simulink subsystem "Distance_from_Speaker"  (R2023b)
settings: Solver=VariableStepAuto  StartTime=0.0  StopTime=10.0  RelTol=1e-3
undefined symbols (not defined in the file): AT_Tag_4_Coordinate_X, AT_Tag_4_Coordinate_Y, AT_Tag_7_Coordinate_X, AT_Tag_7_Coordinate_Y, KF_Vision_Ambiguity_Thresh
libraries: simulink x1
settings Model: Creator=ander  LastModifiedBy=ander

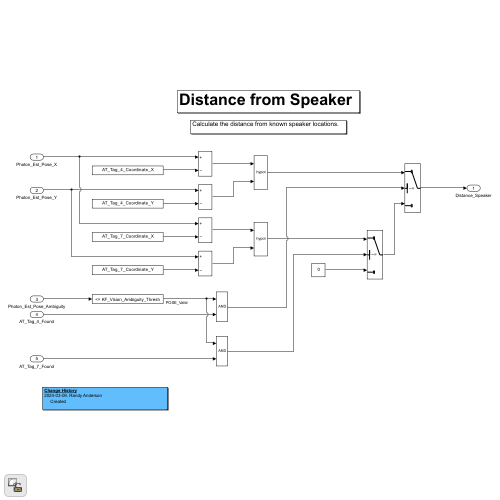
[thumbnail: Simulink's stored preview of the top-level diagram]
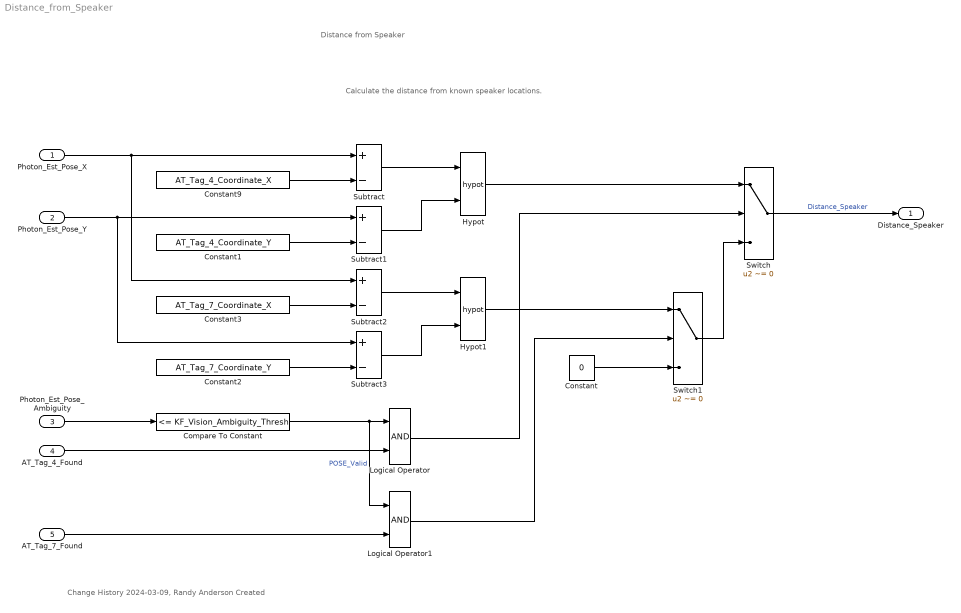
== system Distance_from_Speaker ==
  note: Distance from Speaker
  note: Calculate the distance from known speaker locations.
  note: Change History
      | 2024-03-09, Randy Anderson
      | Created
  Photon_Est_Pose_X : Inport
  Photon_Est_Pose_Y : Inport  Port=2
  Photon_Est_Pose_Ambiguity : Inport  Port=3
  AT_Tag_4_Found : Inport  Port=4
  AT_Tag_7_Found : Inport  Port=5
  Compare To Constant : simulink/Logic and Bit Operations/Compare To Constant  relop=<=  const=KF_Vision_Ambiguity_Thresh  OutDataTypeStr=boolean
  Constant : Constant  Value=0
  Constant1 : Constant  Value=AT_Tag_4_Coordinate_Y
  Constant2 : Constant  Value=AT_Tag_7_Coordinate_Y
  Constant3 : Constant  Value=AT_Tag_7_Coordinate_X
  Constant9 : Constant  Value=AT_Tag_4_Coordinate_X
  Hypot : Math  Operator=hypot
  Hypot1 : Math  Operator=hypot
  Logical Operator : Logic  AllPortsSameDT=off  OutDataTypeStr=boolean
  Logical Operator1 : Logic  AllPortsSameDT=off  OutDataTypeStr=boolean
  Subtract{,1..3} (4 alike) : Sum  Inputs=+-
  Switch : Switch  Criteria=u2 ~= 0  SaturateOnIntegerOverflow=off  InputSameDT=off
  Switch1 : Switch  Criteria=u2 ~= 0  SaturateOnIntegerOverflow=off  InputSameDT=off
  Distance_Speaker : Outport
  wires:
  Photon_Est_Pose_Ambiguity/1 -> Compare To Constant/1
  AT_Tag_4_Found/1 -> Logical Operator/2
  AT_Tag_7_Found/1 -> Logical Operator1/2
  Compare To Constant/1 -> Logical Operator/1, Logical Operator1/1  "POSE_Valid"
  Photon_Est_Pose_X/1 -> Subtract2/1, Subtract/1
  Constant9/1 -> Subtract/2
  Photon_Est_Pose_Y/1 -> Subtract3/1, Subtract1/1
  Constant1/1 -> Subtract1/2
  Constant3/1 -> Subtract2/2
  Constant2/1 -> Subtract3/2
  Subtract/1 -> Hypot/1
  Subtract1/1 -> Hypot/2
  Subtract2/1 -> Hypot1/1
  Subtract3/1 -> Hypot1/2
  Logical Operator/1 -> Switch/2
  Hypot/1 -> Switch/1
  Switch1/1 -> Switch/3
  Hypot1/1 -> Switch1/1
  Logical Operator1/1 -> Switch1/2
  Switch/1 -> Distance_Speaker/1  "Distance_Speaker"
  Constant/1 -> Switch1/3
